simulink model "athree_phase_transestor"  (R2015a)
settings: Solver=ode45  StartTime=0.0  StopTime=0.07  MaxStep=1/10000  RelTol=1e-3
libraries: powerlib x22, simulink_extras x1
settings Model: Creator=Windows 10  LastModifiedBy=Windows 10

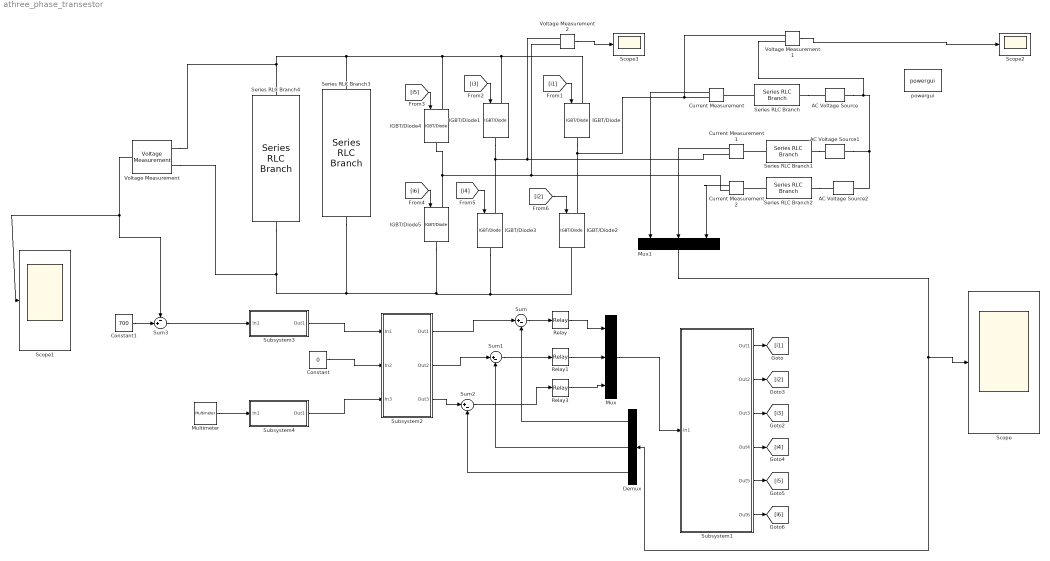
== system athree_phase_transestor ==
  AC Voltage Source : powerlib/Electrical Sources/AC Voltage Source  Amplitude=326.5  Phase=0  Frequency=50  SampleTime=0  Measurements=Voltage
  AC Voltage Source1 : powerlib/Electrical Sources/AC Voltage Source  Amplitude=326.5  Phase=-120  Frequency=50  SampleTime=0  Measurements=Voltage
  AC Voltage Source2 : powerlib/Electrical Sources/AC Voltage Source  Amplitude=326.5  Phase=120  Frequency=50  SampleTime=0  Measurements=Voltage
  Constant : Constant  Value=0
  Constant1 : Constant  Value=700
  Current Measurement : powerlib/Measurements/Current Measurement  PhasorSimulation=off  OutputType=Complex  PSBequivalent=0
  Current Measurement1 : powerlib/Measurements/Current Measurement  PhasorSimulation=off  OutputType=Complex  PSBequivalent=0
  Current Measurement2 : powerlib/Measurements/Current Measurement  PhasorSimulation=off  OutputType=Complex  PSBequivalent=0
  Demux : Demux  Outputs=3
  IGBT/Diode{,1..5} (6 alike) : powerlib/Power Electronics/IGBT//Diode  Ron=1e-3  Rs=1e5  Cs=inf  Measurements=off
  Multimeter : powerlib/Measurements/Multimeter  PhasorSimulation=off  OutputType=Complex  sel=[3 2 1]  L=3  Gain=[1 1 1]  yselected={'Usrc: AC Voltage Source','Usrc: AC Voltage Source1','Usrc: AC Voltage Source2'};  PSBOutputType=1  PSBequivalent=0  AxesSetting=[0,0.1,-100,100]  Display=0  SavedBlockNames=-11
  Mux : Mux  Inputs=3
  Mux1 : Mux  Inputs=3
  Relay : Relay  OnSwitchValue=1  OffSwitchValue=-1  OnOutputValue=-1  OffOutputValue=1
  Relay1 : Relay  OnSwitchValue=1  OffSwitchValue=-1  OnOutputValue=-1  OffOutputValue=1
  Relay3 : Relay  OnSwitchValue=1  OffSwitchValue=-1  OnOutputValue=-1  OffOutputValue=1
  Scope{,1..3} (4 alike) : Scope
      Scope1 settings: YMin=699.875  YMax=700.15
      Scope2 settings: SaveName=ScopeData2
      Scope3 settings: SaveName=ScopeData3
  Series RLC Branch : powerlib/Elements/Series RLC Branch  LConnTagsString=__new0  RConnTagsString=__new0  BranchType=RL  Resistance=0.8  Inductance=1.2e-3  SetiL0=off  InitialCurrent=0  Capacitance=1e-6  Setx0=off  InitialVoltage=0  Measurements=None
  Series RLC Branch1 : powerlib/Elements/Series RLC Branch  LConnTagsString=__new0  RConnTagsString=__new0  BranchType=RL  Resistance=0.8  Inductance=1.2e-3  SetiL0=off  InitialCurrent=0  Capacitance=1e-6  Setx0=off  InitialVoltage=0  Measurements=None
  Series RLC Branch2 : powerlib/Elements/Series RLC Branch  LConnTagsString=__new0  RConnTagsString=__new0  BranchType=RL  Resistance=0.8  Inductance=1.2e-3  SetiL0=off  InitialCurrent=0  Capacitance=1e-6  Setx0=off  InitialVoltage=0  Measurements=None
  Series RLC Branch3 : powerlib/Elements/Series RLC Branch  LConnTagsString=__new0  RConnTagsString=__new0  BranchType=R  Resistance=46.6  Inductance=1e-3  SetiL0=off  InitialCurrent=0  Capacitance=1e-6  Setx0=off  InitialVoltage=0  Measurements=None
  Series RLC Branch4 : powerlib/Elements/Series RLC Branch  LConnTagsString=__new0  RConnTagsString=__new0  BranchType=C  Resistance=1  Inductance=1e-3  SetiL0=off  InitialCurrent=0  Capacitance=1.2/1000  Setx0=on  InitialVoltage=700  Measurements=None
  Subsystem1 : Subsystem
  Subsystem2 : Subsystem
  Subsystem3 : Subsystem
  Subsystem4 : Subsystem
  Sum : Sum  Inputs=|+-
  Sum1 : Sum  Inputs=|+-
  Sum2 : Sum  Inputs=|+-
  Sum3 : Sum  Inputs=-+|
  Voltage Measurement : powerlib/Measurements/Voltage Measurement  PhasorSimulation=off  OutputType=Complex  PSBequivalent=0
  Voltage Measurement1 : powerlib/Measurements/Voltage Measurement  PhasorSimulation=off  OutputType=Complex  PSBequivalent=0
  Voltage Measurement2 : powerlib/Measurements/Voltage Measurement  PhasorSimulation=off  OutputType=Complex  PSBequivalent=0
  powergui : powerlib/powergui  Priority=1  SimulationMode=Continuous  SolverType=Tustin/Backward Euler (TBE)  SampleTime=50e-6  frequency=60  SPID=off  DisableSnubberDevices=off  DisableRonSwitches=off  DisableVfSwitches=off  SwTol=0  DisplayEquations=off  Interpol=off  methode=off  Ts=100  FunctionMessages=off  echomessages=off  HookPort=off  EnableUseOfTLC=off  x0status=blocks  frequencyindice=50  Pbase=100e6  ErrMax=1e-4  Iterations=50  UnitsV=kV  UnitsW=MW  buscounter=0  RestoreLinks=warning  ResistiveCurrentMeasurement=off  Frange=[0:2:500]  Ylog=off  Xlog=on  ShowGrid=off  save=off  variable=ZData  structure=0  ZoomFFT=off  StartTime=0.0  cycles=1  DisplayStyle=1  fundamental=60  FreqAxis=off  MaxFrequency=1000  frequencyindicesteady=1  RmsSteady=1  display=off
  wires:
  Current Measurement2/1 -> Mux1/3
  Current Measurement1/1 -> Mux1/2
  Current Measurement/1 -> Mux1/1
  [i5] -> IGBT/Diode4/1
  [i3] -> IGBT/Diode1/1
  [i1] -> IGBT/Diode/1
  [i6] -> IGBT/Diode5/1
  [i4] -> IGBT/Diode3/1
  [i2] -> IGBT/Diode2/1
  Mux1/1 -> Demux/1, Scope/1
  Demux/1 -> Sum/2
  Demux/2 -> Sum1/2
  Demux/3 -> Sum2/2
  Sum/1 -> Relay/1
  Sum2/1 -> Relay3/1
  Sum1/1 -> Relay1/1
  Relay1/1 -> Mux/2
  Relay/1 -> Mux/1
  Relay3/1 -> Mux/3
  Mux/1 -> Subsystem1/1(In1)
  Subsystem2/1(Out1) -> Sum/1
  Subsystem2/2(Out2) -> Sum1/1
  Subsystem2/3(Out3) -> Sum2/1
  Voltage Measurement/1 -> Sum3/1, Scope1/1
  Sum3/1 -> Subsystem3/1(In1)
  Subsystem3/1(Out1) -> Subsystem2/1(In1)
  Subsystem4/1(Out1) -> Subsystem2/3(In3)
  Constant/1 -> Subsystem2/2(In2)
  Constant1/1 -> Sum3/2
  Multimeter/1 -> Subsystem4/1(In1)
  Subsystem1/1(Out1) -> [i1]
  Subsystem1/3(Out3) -> [i3]
  Subsystem1/2(Out2) -> [i2]
  Subsystem1/4(Out4) -> [i4]
  Subsystem1/5(Out5) -> [i5]
  Subsystem1/6(Out6) -> [i6]
  Voltage Measurement1/1 -> Scope2/1
  Voltage Measurement2/1 -> Scope3/1
  connections:
  AC Voltage Source/LConn1 -- Voltage Measurement1/LConn2 -- AC Voltage Source1/LConn1 -- AC Voltage Source2/LConn1
  Series RLC Branch1/LConn1 -- AC Voltage Source1/RConn1
  Series RLC Branch2/LConn1 -- AC Voltage Source2/RConn1
  Series RLC Branch1/RConn1 -- Current Measurement1/LConn1
  Series RLC Branch2/RConn1 -- Current Measurement2/LConn1
  IGBT/Diode/RConn1 -- Voltage Measurement1/LConn1 -- Current Measurement/RConn1 -- IGBT/Diode2/LConn1
  IGBT/Diode1/RConn1 -- Current Measurement1/RConn1 -- Voltage Measurement2/LConn1 -- IGBT/Diode3/LConn1
  IGBT/Diode4/RConn1 -- Current Measurement2/RConn1 -- Voltage Measurement2/LConn2 -- IGBT/Diode5/LConn1
  IGBT/Diode4/LConn1 -- Voltage Measurement/LConn1 -- Series RLC Branch4/LConn1 -- Series RLC Branch3/LConn1 -- IGBT/Diode/LConn1 -- IGBT/Diode1/LConn1
  IGBT/Diode5/RConn1 -- Series RLC Branch4/RConn1 -- Voltage Measurement/LConn2 -- Series RLC Branch3/RConn1 -- IGBT/Diode3/RConn1 -- IGBT/Diode2/RConn1
  Series RLC Branch/LConn1 -- AC Voltage Source/RConn1
  Series RLC Branch/RConn1 -- Current Measurement/LConn1

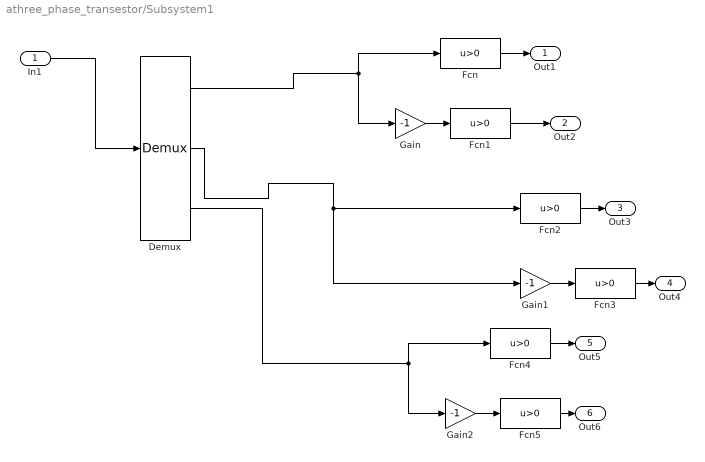
== system athree_phase_transestor/Subsystem1 ==
  In1 : Inport
  Demux : Demux  Outputs=3
  Fcn{,1..5} (6 alike) : Fcn  Expr=u>0
  Gain : Gain  Gain=-1
  Gain1 : Gain  Gain=-1
  Gain2 : Gain  Gain=-1
  Out1 : Outport
  Out2 : Outport  Port=2
  Out3 : Outport  Port=3
  Out4 : Outport  Port=4
  Out5 : Outport  Port=5
  Out6 : Outport  Port=6
  wires:
  In1/1 -> Demux/1
  Gain/1 -> Fcn1/1
  Demux/1 -> Gain/1, Fcn/1
  Gain1/1 -> Fcn3/1
  Demux/2 -> Gain1/1, Fcn2/1
  Gain2/1 -> Fcn5/1
  Demux/3 -> Gain2/1, Fcn4/1
  Fcn1/1 -> Out2/1
  Fcn/1 -> Out1/1
  Fcn2/1 -> Out3/1
  Fcn3/1 -> Out4/1
  Fcn4/1 -> Out5/1
  Fcn5/1 -> Out6/1

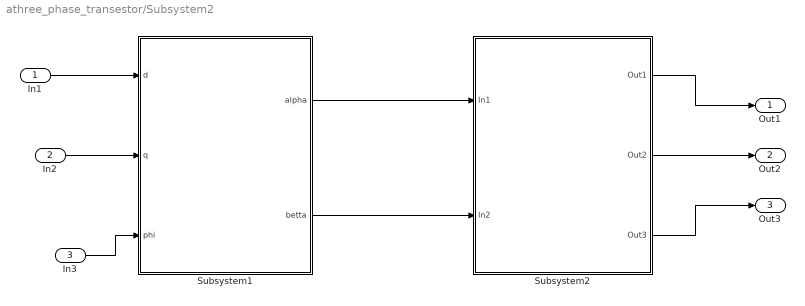
== system athree_phase_transestor/Subsystem2 ==
  In1 : Inport
  In2 : Inport  Port=2
  In3 : Inport  Port=3
  Subsystem1 : Subsystem
  Subsystem2 : Subsystem
  Out1 : Outport
  Out2 : Outport  Port=2
  Out3 : Outport  Port=3
  wires:
  Subsystem2/2(Out2) -> Out2/1
  Subsystem1/1(alpha) -> Subsystem2/1(In1)
  Subsystem2/3(Out3) -> Out3/1
  Subsystem2/1(Out1) -> Out1/1
  In3/1 -> Subsystem1/3(phi)
  In1/1 -> Subsystem1/1(d)
  In2/1 -> Subsystem1/2(q)
  Subsystem1/2(betta) -> Subsystem2/2(In2)

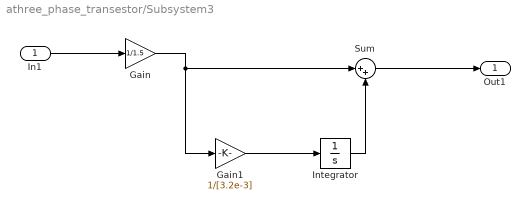
== system athree_phase_transestor/Subsystem3 ==
  In1 : Inport
  Gain : Gain  Gain=1/1.5
  Gain1 : Gain  Gain=1/[3.2e-3]
  Integrator : Integrator
  Sum : Sum  Inputs=|++
  Out1 : Outport
  wires:
  In1/1 -> Gain/1
  Gain/1 -> Sum/1, Gain1/1
  Gain1/1 -> Integrator/1
  Integrator/1 -> Sum/2
  Sum/1 -> Out1/1

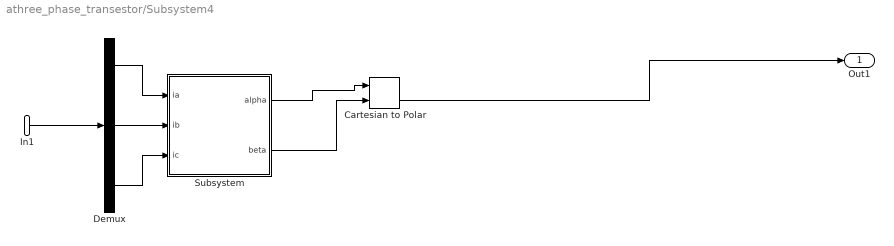
== system athree_phase_transestor/Subsystem4 ==
  In1 : Inport
  Cartesian to Polar : simulink_extras/Transformations/Cartesian to Polar
  Demux : Demux  Outputs=3
  Subsystem : Subsystem
  Out1 : Outport
  wires:
  Subsystem/1(alpha) -> Cartesian to Polar/1
  Subsystem/2(beta) -> Cartesian to Polar/2
  Cartesian to Polar/2 -> Out1/1
  In1/1 -> Demux/1
  Demux/1 -> Subsystem/1(ia)
  Demux/2 -> Subsystem/2(ib)
  Demux/3 -> Subsystem/3(ic)

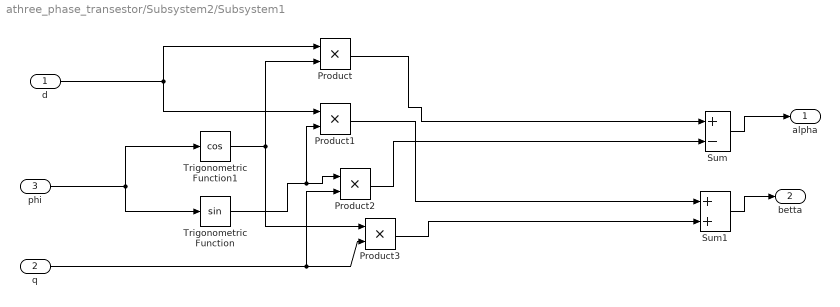
== system athree_phase_transestor/Subsystem2/Subsystem1 ==
  d : Inport
  q : Inport  Port=2
  phi : Inport  Port=3
  Product{,1..3} (4 alike) : Product
  Sum : Sum  Inputs=+-
  Sum1 : Sum
  Trigonometric Function : Trigonometry
  Trigonometric Function1 : Trigonometry  Operator=cos
  alpha : Outport
  betta : Outport  Port=2
  wires:
  Sum/1 -> alpha/1
  Sum1/1 -> betta/1
  phi/1 -> Trigonometric Function/1, Trigonometric Function1/1
  Product/1 -> Sum/1
  Product1/1 -> Sum1/1
  Product2/1 -> Sum/2
  Product3/1 -> Sum1/2
  q/1 -> Product2/2, Product3/2
  Trigonometric Function/1 -> Product1/2, Product2/1
  Trigonometric Function1/1 -> Product3/1, Product/2
  d/1 -> Product1/1, Product/1

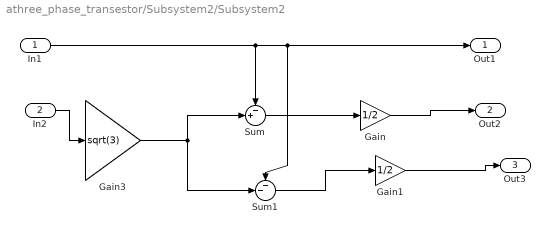
== system athree_phase_transestor/Subsystem2/Subsystem2 ==
  In1 : Inport
  In2 : Inport  Port=2
  Gain : Gain  Gain=1/2
  Gain1 : Gain  Gain=1/2
  Gain3 : Gain  Gain=sqrt(3)
  Sum : Sum  Inputs=-+|
  Sum1 : Sum  Inputs=--|
  Out1 : Outport
  Out2 : Outport  Port=2
  Out3 : Outport  Port=3
  wires:
  Gain/1 -> Out2/1
  Gain1/1 -> Out3/1
  In2/1 -> Gain3/1
  Gain3/1 -> Sum/2, Sum1/2
  In1/1 -> Sum1/1, Out1/1, Sum/1
  Sum/1 -> Gain/1
  Sum1/1 -> Gain1/1

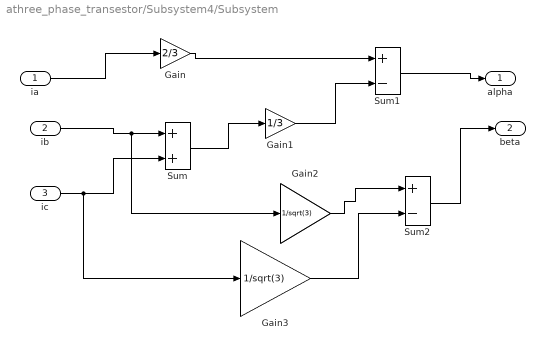
== system athree_phase_transestor/Subsystem4/Subsystem ==
  ia : Inport
  ib : Inport  Port=2
  ic : Inport  Port=3
  Gain : Gain  Gain=2/3
  Gain1 : Gain  Gain=1/3
  Gain2 : Gain  Gain=1/sqrt(3)
  Gain3 : Gain  Gain=1/sqrt(3)
  Sum : Sum
  Sum1 : Sum  Inputs=+-
  Sum2 : Sum  Inputs=+-
  alpha : Outport
  beta : Outport  Port=2
  wires:
  Sum1/1 -> alpha/1
  Sum2/1 -> beta/1
  Gain/1 -> Sum1/1
  Gain1/1 -> Sum1/2
  Sum/1 -> Gain1/1
  ia/1 -> Gain/1
  ib/1 -> Gain2/1, Sum/1
  ic/1 -> Gain3/1, Sum/2
  Gain2/1 -> Sum2/1
  Gain3/1 -> Sum2/2
